simulink library "INT_FanSpd_VD"  (R2016b)
settings: Solver=VariableStepAuto  StartTime=0.0  StopTime=10.0  RelTol=1e-3
settings Model: Creator=xinchangran  LastModifiedBy=xinchangran

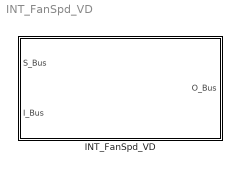
== system INT_FanSpd_VD ==
  INT_FanSpd_VD : Subsystem

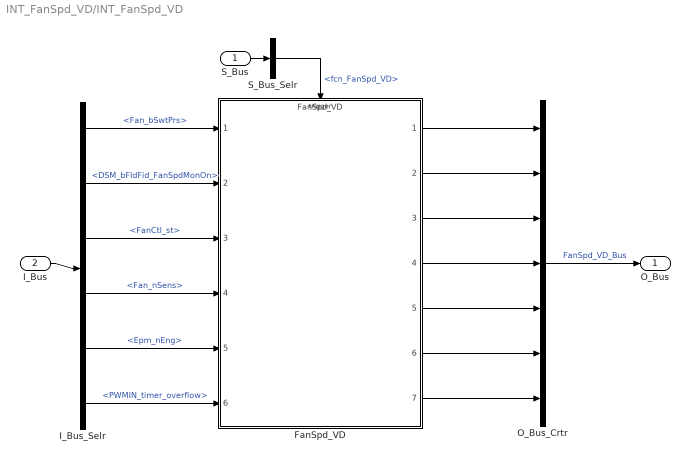
== system INT_FanSpd_VD/INT_FanSpd_VD ==
  S_Bus : Inport
  I_Bus : Inport  Port=2
  FanSpd_VD : ModelReference  ModelNameDialog=FanSpd_VD  SimulationMode=Normal  ModelReferenceVersion=1.103  TriggerPortName=function  TriggerPortTriggerType=function-call  TriggerPortStatesWhenEnabling=held
  I_Bus_Selr : BusSelector  OutputSignals=Fan_bSwtPrs,DSM_bFIdFid_FanSpdMonOn,FanCtl_st,Fan_nSens,Epm_nEng,PWMIN_timer_overflow
  O_Bus_Crtr : BusCreator  Inputs=7
  S_Bus_Selr : BusSelector  OutputSignals=fcn_FanSpd_VD
  O_Bus : Outport
  wires:
  S_Bus_Selr/1 -> FanSpd_VD/Trigger  "<fcn_FanSpd_VD>"
  S_Bus/1 -> S_Bus_Selr/1
  I_Bus/1 -> I_Bus_Selr/1
  I_Bus_Selr/1 -> FanSpd_VD/1  "<Fan_bSwtPrs>"
  I_Bus_Selr/2 -> FanSpd_VD/2  "<DSM_bFIdFid_FanSpdMonOn>"
  I_Bus_Selr/3 -> FanSpd_VD/3  "<FanCtl_st>"
  I_Bus_Selr/4 -> FanSpd_VD/4  "<Fan_nSens>"
  I_Bus_Selr/5 -> FanSpd_VD/5  "<Epm_nEng>"
  I_Bus_Selr/6 -> FanSpd_VD/6  "<PWMIN_timer_overflow>"
  O_Bus_Crtr/1 -> O_Bus/1  "FanSpd_VD_Bus"
  FanSpd_VD/1 -> O_Bus_Crtr/1
  FanSpd_VD/2 -> O_Bus_Crtr/2
  FanSpd_VD/3 -> O_Bus_Crtr/3
  FanSpd_VD/4 -> O_Bus_Crtr/4
  FanSpd_VD/5 -> O_Bus_Crtr/5
  FanSpd_VD/6 -> O_Bus_Crtr/6
  FanSpd_VD/7 -> O_Bus_Crtr/7
